simulink model "PTTransmCU"  (Simulink 7.5)
settings: Solver=ode45  StartTime=0.0  StopTime=inf  RelTol=1e-3
libraries: simulink x12, CarMaker4SL x1
(part 2 of 3)

== system PTTransmCU/CarMaker/IPG Vehicle/CarAndTrailer/Forces/Vehicle Forces ==
  Sync_In : Inport  OutDataType=sfix(16)  OutScaling=2^0
  Bus Creator1 : BusCreator  Inputs=12
  Bus Creator5 : BusCreator  Inputs=13
  Bus Creator8 : BusCreator  Inputs=16
  Demux : Demux  Outputs=16
  Demux1 : Demux  Outputs=12
  Demux5 : Demux  Outputs=13
  Forces : S-Function  FunctionName=CM_Sfun  Parameters='Forces'  EnableBusSupport=off
  Sync_Out : Outport  OutDataType=sfix(16)  OutScaling=2^0
  Car.Virtual : Outport  Port=2  OutDataType=sfix(16)  OutScaling=2^0
  Car.Aero : Outport  Port=3  OutDataType=sfix(16)  OutScaling=2^0
  Car.Load : Outport  Port=4  OutDataType=sfix(16)  OutScaling=2^0
  wires:
  Demux5/7 -> Bus Creator5/7  "car Aero vRes_1 z"
  Demux5/6 -> Bus Creator5/6  "car Aero vRes_1 y"
  Demux5/5 -> Bus Creator5/5  "car Aero vRes_1 x"
  Demux5/4 -> Bus Creator5/4  "Vehicle Wind_vel_0 z"
  Demux5/3 -> Bus Creator5/3  "Vehicle Wind_vel_0 y"
  Demux5/2 -> Bus Creator5/2  "Vehicle Wind_vel_0 x"
  Demux5/1 -> Bus Creator5/1  "Vehicle sRoadAero"
  Demux5/8 -> Bus Creator5/8  "car Aero Frc_1 x"
  Demux5/9 -> Bus Creator5/9  "car Aero Frc_1 y"
  Demux5/10 -> Bus Creator5/10  "car Aero Frc_1 z"
  Demux5/13 -> Bus Creator5/13  "car Aero Trq_1 z"
  Demux5/12 -> Bus Creator5/12  "car Aero Trq_1 y"
  Demux5/11 -> Bus Creator5/11  "car Aero Trq_1 x"
  Forces/4 -> Demux/1
  Demux/12 -> Bus Creator8/12  "Car Load_2 tz"
  Demux/11 -> Bus Creator8/11  "Car Load_2 ty"
  Demux/10 -> Bus Creator8/10  "Car Load_2 tx"
  Demux/9 -> Bus Creator8/9  "Car Load_2 mass"
  Demux/8 -> Bus Creator8/8  "Car Load_1 tz"
  Demux/7 -> Bus Creator8/7  "Car Load_1 ty"
  Demux/6 -> Bus Creator8/6  "Car Load_1 tx"
  Demux/5 -> Bus Creator8/5  "Car Load_1 mass"
  Demux/4 -> Bus Creator8/4  "Car Load_0 tz"
  Demux/3 -> Bus Creator8/3  "Car Load_0 ty"
  Demux/2 -> Bus Creator8/2  "Car Load_0 tx"
  Demux/1 -> Bus Creator8/1  "Car Load_0 mass"
  Bus Creator8/1 -> Car.Load/1
  Bus Creator1/1 -> Car.Virtual/1
  Forces/2 -> Demux1/1
  Forces/3 -> Demux5/1
  Demux1/3 -> Bus Creator1/3  "Car Virtual Frc_1 z"
  Demux1/2 -> Bus Creator1/2  "Car Virtual Frc_1 y"
  Demux1/1 -> Bus Creator1/1  "Car Virtual Frc_1 x"
  Bus Creator5/1 -> Car.Aero/1
  Forces/1 -> Sync_Out/1
  Sync_In/1 -> Forces/1
  Demux1/4 -> Bus Creator1/4  "Car Virtual Frc_0 x"
  Demux1/5 -> Bus Creator1/5  "Car Virtual Frc_0 y"
  Demux1/6 -> Bus Creator1/6  "Car Virtual Frc_0 z"
  Demux1/7 -> Bus Creator1/7  "Car Virtual Trq_1 x"
  Demux1/8 -> Bus Creator1/8  "Car Virtual Trq_1 y"
  Demux1/9 -> Bus Creator1/9  "Car Virtual Trq_1 z"
  Demux1/10 -> Bus Creator1/10  "Car Virtual Trq_0 x"
  Demux1/11 -> Bus Creator1/11  "Car Virtual Trq_0 y"
  Demux1/12 -> Bus Creator1/12  "Car Virtual Trq_0 z"
  Demux/13 -> Bus Creator8/13  "Car Load_3 mass"
  Demux/14 -> Bus Creator8/14  "Car Load_3 tx"
  Demux/15 -> Bus Creator8/15  "Car Load_3 ty"
  Demux/16 -> Bus Creator8/16  "Car Load_3 tz"

== system PTTransmCU/CarMaker/IPG Vehicle/CarAndTrailer/Trailer/CreateBus Car.Hitch.FrcTrq ==
  In1 : Inport  OutDataType=sfix(16)  OutScaling=2^0
  Bus Creator7 : BusCreator  Inputs=6
  Demux7 : Demux  Outputs=6
  Car.Hitch.FrcTrq : Outport  OutDataType=sfix(16)  OutScaling=2^0
  wires:
  Demux7/1 -> Bus Creator7/1  "Car Hitch Frc2Car x"
  Demux7/2 -> Bus Creator7/2  "Car Hitch Frc2Car y"
  Demux7/3 -> Bus Creator7/3  "Car Hitch Frc2Car z"
  Demux7/4 -> Bus Creator7/4  "Car Hitch Trq2Car x"
  Demux7/5 -> Bus Creator7/5  "Car Hitch Trq2Car y"
  Demux7/6 -> Bus Creator7/6  "Car Hitch Trq2Car z"
  Bus Creator7/1 -> Car.Hitch.FrcTrq/1
  In1/1 -> Demux7/1

== system PTTransmCU/CarMaker/IPG Vehicle/CarAndTrailer/Trailer/CreateBus Vhcl.Motion ==
  In1 : Inport  OutDataType=sfix(16)  OutScaling=2^0
  Demux1 : Demux  Outputs=16
  Mux1 : Mux  Inputs=16
  Out1 : Outport  OutDataType=sfix(16)  OutScaling=2^0
  wires:
  Mux1/1 -> Out1/1
  In1/1 -> Demux1/1
  Demux1/16 -> Mux1/16  "Vhcl YawAcc"
  Demux1/15 -> Mux1/15  "Vhcl YawRate"
  Demux1/14 -> Mux1/14  "Vhcl Yaw"
  Demux1/13 -> Mux1/13  "Vhcl PitchAcc"
  Demux1/12 -> Mux1/12  "Vhcl PitchVel"
  Demux1/11 -> Mux1/11  "Vhcl Pitch"
  Demux1/10 -> Mux1/10  "Vhcl RollAcc"
  Demux1/9 -> Mux1/9  "Vhcl RollVel"
  Demux1/8 -> Mux1/8  "Vhcl Roll"
  Demux1/7 -> Mux1/7  "Vhcl Hitch_Pos z"
  Demux1/6 -> Mux1/6  "Vhcl Hitch_Pos y"
  Demux1/5 -> Mux1/5  "Vhcl Hitch_Pos x"
  Demux1/4 -> Mux1/4  "Vhcl sRoadAero"
  Demux1/3 -> Mux1/3  "Vhcl sRoad"
  Demux1/2 -> Mux1/2  "Vhcl Distance"
  Demux1/1 -> Mux1/1  "Vhcl v"

== system PTTransmCU/CarMaker/IPG Vehicle/CarAndTrailer/Trailer/CreateBus Vhcl.PoI ==
  In1 : Inport  OutDataType=sfix(16)  OutScaling=2^0
  Bus Creator3 : BusCreator  Inputs=18
  Demux3 : Demux  Outputs=18
  Out1 : Outport  OutDataType=sfix(16)  OutScaling=2^0
  wires:
  Demux3/1 -> Bus Creator3/1  "Vhcl PoI_Pos x"
  Bus Creator3/1 -> Out1/1
  In1/1 -> Demux3/1
  Demux3/2 -> Bus Creator3/2  "Vhcl PoI_Pos y"
  Demux3/3 -> Bus Creator3/3  "Vhcl PoI_Pos z"
  Demux3/4 -> Bus Creator3/4  "Vhcl PoI_Vel x"
  Demux3/5 -> Bus Creator3/5  "Vhcl PoI_Vel y"
  Demux3/6 -> Bus Creator3/6  "Vhcl PoI_Vel z"
  Demux3/7 -> Bus Creator3/7  "Vhcl PoI_Acc x"
  Demux3/8 -> Bus Creator3/8  "Vhcl PoI_Acc y"
  Demux3/9 -> Bus Creator3/9  "Vhcl PoI_Acc z"
  Demux3/10 -> Bus Creator3/10  "Vhcl PoI_Vel_1 x"
  Demux3/11 -> Bus Creator3/11  "Vhcl PoI_Vel_1 y"
  Demux3/12 -> Bus Creator3/12  "Vhcl PoI_Vel_1 z"
  Demux3/13 -> Bus Creator3/13  "Vhcl PoI_Acc_1 x"
  Demux3/14 -> Bus Creator3/14  "Vhcl PoI_Acc_1 y"
  Demux3/15 -> Bus Creator3/15  "Vhcl PoI_Acc_1 z"
  Demux3/16 -> Bus Creator3/16  "Vhcl PoI_GCS Long"
  Demux3/17 -> Bus Creator3/17  "Vhcl PoI_GCS Lat"
  Demux3/18 -> Bus Creator3/18  "Vhcl PoI_GCS Elev"

== system PTTransmCU/CarMaker/IPG Vehicle/CarAndTrailer/Trailer/CreateBus Vhcl.Steering ==
  In1 : Inport  OutDataType=sfix(16)  OutScaling=2^0
  Bus Creator3 : BusCreator
  Demux : Demux
  Out1 : Outport  OutDataType=sfix(16)  OutScaling=2^0
  wires:
  In1/1 -> Demux/1
  Demux/4 -> Bus Creator3/4  "Vhcl Steering Trq"
  Demux/2 -> Bus Creator3/2  "Vhcl Steering AngVel"
  Demux/3 -> Bus Creator3/3  "Vhcl Steering AngAcc"
  Demux/1 -> Bus Creator3/1  "Vhcl Steering Ang"
  Bus Creator3/1 -> Out1/1

== system PTTransmCU/CarMaker/IPG Vehicle/CarAndTrailer/Trailer/CreateBus Vhcl.Wheel.FL ==
  In1 : Inport  OutDataType=sfix(16)  OutScaling=2^0
  Bus Creator3 : BusCreator  Inputs=14
  Demux3 : Demux  Outputs=14
  Out1 : Outport  OutDataType=sfix(16)  OutScaling=2^0
  wires:
  Demux3/1 -> Bus Creator3/1  "Vhcl Wheel FL t x"
  Bus Creator3/1 -> Out1/1
  In1/1 -> Demux3/1
  Demux3/2 -> Bus Creator3/2  "Vhcl Wheel FL t y"
  Demux3/3 -> Bus Creator3/3  "Vhcl Wheel FL t z"
  Demux3/4 -> Bus Creator3/4  "Vhcl Wheel FL r_zxy x"
  Demux3/5 -> Bus Creator3/5  "Vhcl Wheel FL r_zxy y"
  Demux3/6 -> Bus Creator3/6  "Vhcl Wheel FL r_zxy z"
  Demux3/7 -> Bus Creator3/7  "Vhcl Wheel FL Fx"
  Demux3/8 -> Bus Creator3/8  "Vhcl Wheel FL Fy"
  Demux3/9 -> Bus Creator3/9  "Vhcl Wheel FL Fz"
  Demux3/10 -> Bus Creator3/10  "Vhcl Wheel FL vBelt"
  Demux3/11 -> Bus Creator3/11  "Vhcl Wheel FL LongSlip"
  Demux3/12 -> Bus Creator3/12  "Vhcl Wheel FL SideSlip"
  Demux3/13 -> Bus Creator3/13  "Vhcl Wheel FL Trq_T2W"
  Demux3/14 -> Bus Creator3/14  "Vhcl Wheel FL Trq_WhlBearing"

== system PTTransmCU/CarMaker/IPG Vehicle/CarAndTrailer/Trailer/CreateBus Vhcl.Wheel.FR ==
  In1 : Inport  OutDataType=sfix(16)  OutScaling=2^0
  Bus Creator3 : BusCreator  Inputs=14
  Demux3 : Demux  Outputs=14
  Out1 : Outport  OutDataType=sfix(16)  OutScaling=2^0
  wires:
  Demux3/1 -> Bus Creator3/1  "Vhcl Wheel FR t x"
  Bus Creator3/1 -> Out1/1
  In1/1 -> Demux3/1
  Demux3/2 -> Bus Creator3/2  "Vhcl Wheel FR t y"
  Demux3/3 -> Bus Creator3/3  "Vhcl Wheel FR t z"
  Demux3/4 -> Bus Creator3/4  "Vhcl Wheel FR r_zxy x"
  Demux3/5 -> Bus Creator3/5  "Vhcl Wheel FR r_zxy y"
  Demux3/6 -> Bus Creator3/6  "Vhcl Wheel FR r_zxy z"
  Demux3/7 -> Bus Creator3/7  "Vhcl Wheel FR Fx"
  Demux3/8 -> Bus Creator3/8  "Vhcl Wheel FR Fy"
  Demux3/9 -> Bus Creator3/9  "Vhcl Wheel FR Fz"
  Demux3/10 -> Bus Creator3/10  "Vhcl Wheel FR vBelt"
  Demux3/11 -> Bus Creator3/11  "Vhcl Wheel FR LongSlip"
  Demux3/12 -> Bus Creator3/12  "Vhcl Wheel FR SideSlip"
  Demux3/13 -> Bus Creator3/13  "Vhcl Wheel FR Trq_T2W"
  Demux3/14 -> Bus Creator3/14  "Vhcl Wheel FR Trq_WhlBearing"

== system PTTransmCU/CarMaker/IPG Vehicle/CarAndTrailer/Trailer/CreateBus Vhcl.Wheel.RL ==
  In1 : Inport  OutDataType=sfix(16)  OutScaling=2^0
  Bus Creator3 : BusCreator  Inputs=14
  Demux3 : Demux  Outputs=14
  Out1 : Outport  OutDataType=sfix(16)  OutScaling=2^0
  wires:
  Demux3/1 -> Bus Creator3/1  "Vhcl Wheel RL t x"
  Bus Creator3/1 -> Out1/1
  In1/1 -> Demux3/1
  Demux3/2 -> Bus Creator3/2  "Vhcl Wheel RL t y"
  Demux3/3 -> Bus Creator3/3  "Vhcl Wheel RL t z"
  Demux3/4 -> Bus Creator3/4  "Vhcl Wheel RL r_zxy x"
  Demux3/5 -> Bus Creator3/5  "Vhcl Wheel RL r_zxy y"
  Demux3/6 -> Bus Creator3/6  "Vhcl Wheel RL r_zxy z"
  Demux3/7 -> Bus Creator3/7  "Vhcl Wheel RL Fx"
  Demux3/8 -> Bus Creator3/8  "Vhcl Wheel RL Fy"
  Demux3/9 -> Bus Creator3/9  "Vhcl Wheel RL Fz"
  Demux3/10 -> Bus Creator3/10  "Vhcl Wheel RL vBelt"
  Demux3/11 -> Bus Creator3/11  "Vhcl Wheel RL LongSlip"
  Demux3/12 -> Bus Creator3/12  "Vhcl Wheel RL SideSlip"
  Demux3/13 -> Bus Creator3/13  "Vhcl Wheel RL Trq_T2W"
  Demux3/14 -> Bus Creator3/14  "Vhcl Wheel RL Trq_WhlBearing"

== system PTTransmCU/CarMaker/IPG Vehicle/CarAndTrailer/Trailer/CreateBus Vhcl.Wheel.RR ==
  In1 : Inport  OutDataType=sfix(16)  OutScaling=2^0
  Bus Creator3 : BusCreator  Inputs=14
  Demux3 : Demux  Outputs=14
  Out1 : Outport  OutDataType=sfix(16)  OutScaling=2^0
  wires:
  Demux3/1 -> Bus Creator3/1  "Vhcl Wheel RR t x"
  Bus Creator3/1 -> Out1/1
  In1/1 -> Demux3/1
  Demux3/2 -> Bus Creator3/2  "Vhcl Wheel RR t y"
  Demux3/3 -> Bus Creator3/3  "Vhcl Wheel RR t z"
  Demux3/4 -> Bus Creator3/4  "Vhcl Wheel RR r_zxy x"
  Demux3/5 -> Bus Creator3/5  "Vhcl Wheel RR r_zxy y"
  Demux3/6 -> Bus Creator3/6  "Vhcl Wheel RR r_zxy z"
  Demux3/7 -> Bus Creator3/7  "Vhcl Wheel RR Fx"
  Demux3/8 -> Bus Creator3/8  "Vhcl Wheel RR Fy"
  Demux3/9 -> Bus Creator3/9  "Vhcl Wheel RR Fz"
  Demux3/10 -> Bus Creator3/10  "Vhcl Wheel RR vBelt"
  Demux3/11 -> Bus Creator3/11  "Vhcl Wheel RR LongSlip"
  Demux3/12 -> Bus Creator3/12  "Vhcl Wheel RR SideSlip"
  Demux3/13 -> Bus Creator3/13  "Vhcl Wheel RR Trq_T2W"
  Demux3/14 -> Bus Creator3/14  "Vhcl Wheel RR Trq_WhlBearing"

== system PTTransmCU/CarMaker/IPG Vehicle/PowerTrain/TCU Example/CreateBus TCU ClutchOut ==
  In : Inport
  BusCreator : BusCreator  Inputs=1
  Demux : Demux  Outputs=1
  Out : Outport
  wires:
  In/1 -> Demux/1
  BusCreator/1 -> Out/1
  Demux/1 -> BusCreator/1  "TCU ClutchOut Pos"

== system PTTransmCU/CarMaker/IPG Vehicle/PowerTrain/TCU Example/CreateBus TCU GearBoxM_Out0 ==
  In : Inport
  BusCreator : BusCreator
  Demux : Demux
  Out : Outport
  wires:
  In/1 -> Demux/1
  BusCreator/1 -> Out/1
  Demux/1 -> BusCreator/1  "TCU GearBoxM_Out0 GearNoTrg"
  Demux/2 -> BusCreator/2  "TCU GearBoxM_Out0 set_ParkBrake"
  Demux/3 -> BusCreator/3  "TCU GearBoxM_Out0 Trq_in_off"
  Demux/4 -> BusCreator/4  "TCU GearBoxM_Out0 Clutch Pos"

== system PTTransmCU/CarMaker/IPG Vehicle/PowerTrain/TCU Example/CreateBus TCU GearBoxM_Out1 ==
  In : Inport
  BusCreator : BusCreator
  Demux : Demux
  Out : Outport
  wires:
  In/1 -> Demux/1
  BusCreator/1 -> Out/1
  Demux/1 -> BusCreator/1  "TCU GearBoxM_Out1 GearNoTrg"
  Demux/2 -> BusCreator/2  "TCU GearBoxM_Out1 set_ParkBrake"
  Demux/3 -> BusCreator/3  "TCU GearBoxM_Out1 Trq_in_off"
  Demux/4 -> BusCreator/4  "TCU GearBoxM_Out1 Clutch Pos"

== system PTTransmCU/CarMaker/IPG Vehicle/PowerTrain/TCU Example/CreateBus TCU GearBoxM_Out2 ==
  In : Inport
  BusCreator : BusCreator
  Demux : Demux
  Out : Outport
  wires:
  In/1 -> Demux/1
  BusCreator/1 -> Out/1
  Demux/1 -> BusCreator/1  "TCU GearBoxM_Out2 GearNoTrg"
  Demux/2 -> BusCreator/2  "TCU GearBoxM_Out2 set_ParkBrake"
  Demux/3 -> BusCreator/3  "TCU GearBoxM_Out2 Trq_in_off"
  Demux/4 -> BusCreator/4  "TCU GearBoxM_Out2 Clutch Pos"

== system PTTransmCU/CarMaker/IPG Vehicle/PowerTrain/TCU Example/CreateBus TCU GearBoxM_Out3 ==
  In : Inport
  BusCreator : BusCreator
  Demux : Demux
  Out : Outport
  wires:
  In/1 -> Demux/1
  BusCreator/1 -> Out/1
  Demux/1 -> BusCreator/1  "TCU GearBoxM_Out3 GearNoTrg"
  Demux/2 -> BusCreator/2  "TCU GearBoxM_Out3 set_ParkBrake"
  Demux/3 -> BusCreator/3  "TCU GearBoxM_Out3 Trq_in_off"
  Demux/4 -> BusCreator/4  "TCU GearBoxM_Out3 Clutch Pos"

== system PTTransmCU/CarMaker/IPG Vehicle/PowerTrain/TCU Example/CreateBus TCU GearBoxOut ==
  In : Inport
  BusCreator : BusCreator
  Demux : Demux
  Out : Outport
  wires:
  In/1 -> Demux/1
  BusCreator/1 -> Out/1
  Demux/1 -> BusCreator/1  "TCU GearBoxOut GearNoTrg"
  Demux/2 -> BusCreator/2  "TCU GearBoxOut set_ParkBrake"
  Demux/3 -> BusCreator/3  "TCU GearBoxOut Trq_in_off"
  Demux/4 -> BusCreator/4  "TCU GearBoxOut Clutch Pos"

== system PTTransmCU/CarMaker/IPG Vehicle/PowerTrain/TCU Example/CreateBus TCU Status ==
  In : Inport
  BusCreator : BusCreator  Inputs=1
  Demux : Demux  Outputs=1
  Out : Outport
  wires:
  In/1 -> Demux/1
  BusCreator/1 -> Out/1
  Demux/1 -> BusCreator/1  "TCU_Out Status"

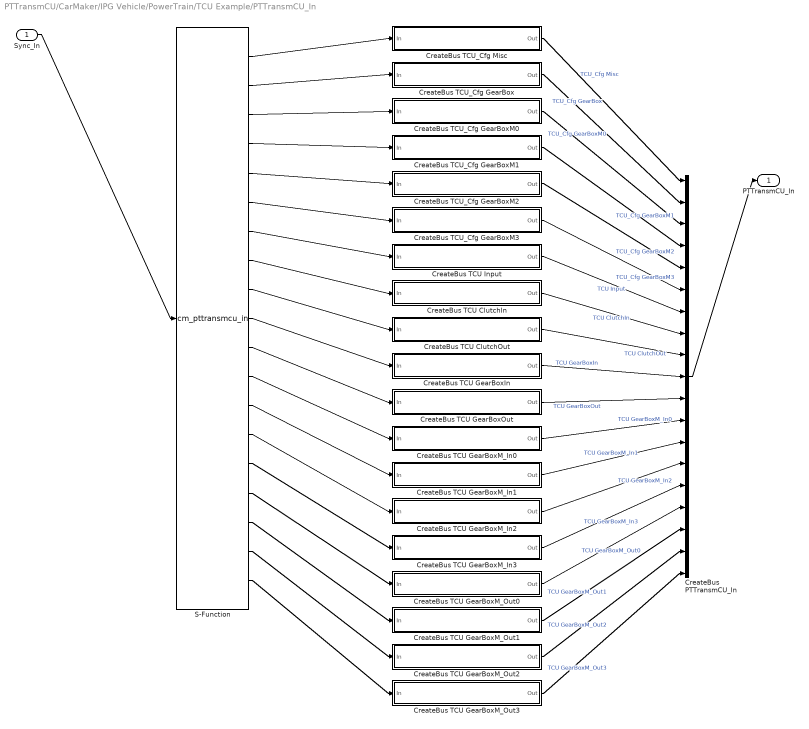
== system PTTransmCU/CarMaker/IPG Vehicle/PowerTrain/TCU Example/PTTransmCU_In ==
  Sync_In : Inport
  CreateBus PTTransmCU_In : BusCreator  Inputs=19
  CreateBus TCU ClutchIn : Subsystem
  CreateBus TCU ClutchOut : Subsystem
  CreateBus TCU GearBoxIn : Subsystem
  CreateBus TCU GearBoxM_In0 : Subsystem
  CreateBus TCU GearBoxM_In1 : Subsystem
  CreateBus TCU GearBoxM_In2 : Subsystem
  CreateBus TCU GearBoxM_In3 : Subsystem
  CreateBus TCU GearBoxM_Out0 : Subsystem
  CreateBus TCU GearBoxM_Out1 : Subsystem
  CreateBus TCU GearBoxM_Out2 : Subsystem
  CreateBus TCU GearBoxM_Out3 : Subsystem
  CreateBus TCU GearBoxOut : Subsystem
  CreateBus TCU Input : Subsystem
  CreateBus TCU_Cfg GearBox : Subsystem
  CreateBus TCU_Cfg GearBoxM0 : Subsystem
  CreateBus TCU_Cfg GearBoxM1 : Subsystem
  CreateBus TCU_Cfg GearBoxM2 : Subsystem
  CreateBus TCU_Cfg GearBoxM3 : Subsystem
  CreateBus TCU_Cfg Misc : Subsystem
  S-Function : S-Function  FunctionName=cm_pttransmcu_in  EnableBusSupport=off
  PTTransmCU_In : Outport
  wires:
  Sync_In/1 -> S-Function/1
  CreateBus PTTransmCU_In/1 -> PTTransmCU_In/1
  S-Function/1 -> CreateBus TCU_Cfg Misc/1(In)
  CreateBus TCU_Cfg Misc/1(Out) -> CreateBus PTTransmCU_In/1  "TCU_Cfg Misc"
  S-Function/2 -> CreateBus TCU_Cfg GearBox/1(In)
  CreateBus TCU_Cfg GearBox/1(Out) -> CreateBus PTTransmCU_In/2  "TCU_Cfg GearBox"
  S-Function/3 -> CreateBus TCU_Cfg GearBoxM0/1(In)
  CreateBus TCU_Cfg GearBoxM0/1(Out) -> CreateBus PTTransmCU_In/3  "TCU_Cfg GearBoxM0"
  S-Function/4 -> CreateBus TCU_Cfg GearBoxM1/1(In)
  CreateBus TCU_Cfg GearBoxM1/1(Out) -> CreateBus PTTransmCU_In/4  "TCU_Cfg GearBoxM1"
  S-Function/5 -> CreateBus TCU_Cfg GearBoxM2/1(In)
  CreateBus TCU_Cfg GearBoxM2/1(Out) -> CreateBus PTTransmCU_In/5  "TCU_Cfg GearBoxM2"
  S-Function/6 -> CreateBus TCU_Cfg GearBoxM3/1(In)
  CreateBus TCU_Cfg GearBoxM3/1(Out) -> CreateBus PTTransmCU_In/6  "TCU_Cfg GearBoxM3"
  S-Function/7 -> CreateBus TCU Input/1(In)
  CreateBus TCU Input/1(Out) -> CreateBus PTTransmCU_In/7  "TCU Input"
  S-Function/8 -> CreateBus TCU ClutchIn/1(In)
  CreateBus TCU ClutchIn/1(Out) -> CreateBus PTTransmCU_In/8  "TCU ClutchIn"
  S-Function/9 -> CreateBus TCU ClutchOut/1(In)
  CreateBus TCU ClutchOut/1(Out) -> CreateBus PTTransmCU_In/9  "TCU ClutchOut"
  S-Function/10 -> CreateBus TCU GearBoxIn/1(In)
  CreateBus TCU GearBoxIn/1(Out) -> CreateBus PTTransmCU_In/10  "TCU GearBoxIn"
  S-Function/11 -> CreateBus TCU GearBoxOut/1(In)
  CreateBus TCU GearBoxOut/1(Out) -> CreateBus PTTransmCU_In/11  "TCU GearBoxOut"
  S-Function/12 -> CreateBus TCU GearBoxM_In0/1(In)
  CreateBus TCU GearBoxM_In0/1(Out) -> CreateBus PTTransmCU_In/12  "TCU GearBoxM_In0"
  S-Function/13 -> CreateBus TCU GearBoxM_In1/1(In)
  CreateBus TCU GearBoxM_In1/1(Out) -> CreateBus PTTransmCU_In/13  "TCU GearBoxM_In1"
  S-Function/14 -> CreateBus TCU GearBoxM_In2/1(In)
  CreateBus TCU GearBoxM_In2/1(Out) -> CreateBus PTTransmCU_In/14  "TCU GearBoxM_In2"
  S-Function/15 -> CreateBus TCU GearBoxM_In3/1(In)
  CreateBus TCU GearBoxM_In3/1(Out) -> CreateBus PTTransmCU_In/15  "TCU GearBoxM_In3"
  S-Function/16 -> CreateBus TCU GearBoxM_Out0/1(In)
  CreateBus TCU GearBoxM_Out0/1(Out) -> CreateBus PTTransmCU_In/16  "TCU GearBoxM_Out0"
  S-Function/17 -> CreateBus TCU GearBoxM_Out1/1(In)
  CreateBus TCU GearBoxM_Out1/1(Out) -> CreateBus PTTransmCU_In/17  "TCU GearBoxM_Out1"
  S-Function/18 -> CreateBus TCU GearBoxM_Out2/1(In)
  CreateBus TCU GearBoxM_Out2/1(Out) -> CreateBus PTTransmCU_In/18  "TCU GearBoxM_Out2"
  S-Function/19 -> CreateBus TCU GearBoxM_Out3/1(In)
  CreateBus TCU GearBoxM_Out3/1(Out) -> CreateBus PTTransmCU_In/19  "TCU GearBoxM_Out3"

== system PTTransmCU/CarMaker/IPG Vehicle/PowerTrain/TCU Example/PTTransmCU_Out ==
  TCU Status : Inport
  TCU ClutchOut : Inport  Port=2
  TCU GearBoxOut : Inport  Port=3
  TCU GearBoxM_Out0 : Inport  Port=4
  TCU GearBoxM_Out1 : Inport  Port=5
  TCU GearBoxM_Out2 : Inport  Port=6
  TCU GearBoxM_Out3 : Inport  Port=7
  S-Function : S-Function  FunctionName=cm_pttransmcu_out  EnableBusSupport=off
  wires:
  TCU Status/1 -> S-Function/1
  TCU ClutchOut/1 -> S-Function/2
  TCU GearBoxOut/1 -> S-Function/3
  TCU GearBoxM_Out0/1 -> S-Function/4
  TCU GearBoxM_Out1/1 -> S-Function/5
  TCU GearBoxM_Out2/1 -> S-Function/6
  TCU GearBoxM_Out3/1 -> S-Function/7

== system PTTransmCU/CarMaker/IPG Vehicle/PowerTrain/TCU Example/TCU Example ==
  note: PTTransmCU model MyTransmCU example, that only works with
      | the 'Generic' powertrain and the 'Manual' gearbox.
  TCUIn : Inport  OutDataType=sfix(16)  OutScaling=2^0
  Bus Creator : BusCreator  Inputs=2
  Bus Selector : BusSelector  OutputSignals=TCU GearBoxIn GearNoTrg
  Bus Selector1 : BusSelector  OutputSignals=TCU Input.TCU Ignition,TCU GearBoxIn.TCU GearBoxIn GearNo,TCU GearBoxOut,TCU ClutchOut,TCU_Cfg GearBox.TCU_Cfg GearBox nFGears,TCU_Cfg GearBox.TCU_Cfg GearBox nBGears
  Bus Selector2 : BusSelector  OutputSignals=TCU GearBoxIn GearNoTrg,TCU GearBoxIn set_ParkBrake,TCU GearBoxIn Clutch Pos
  Don't do anything : Subsystem  TreatAsAtomicUnit=on
  If : If  NumInputs=3  IfExpression=~u1  ElseIfExpressions=u2 == u3
  If Action Subsystem2 : Subsystem  TreatAsAtomicUnit=on
  Merge1 : Merge  Inputs=3
  Merge2 : Merge  Inputs=3  InitialOutput=0
  Retrun Zero : Subsystem  TreatAsAtomicUnit=on
  ClutchOut.Pos : Outport  OutDataType=sfix(16)  OutScaling=2^0
  GearBoxOut.GearNoTrg : Outport  Port=2  OutDataType=sfix(16)  OutScaling=2^0
  GearBoxOut.set_ParkBrake : Outport  Port=3  OutDataType=sfix(16)  OutScaling=2^0
  GearBoxOut.Clutch.Pos : Outport  Port=4  OutDataType=sfix(16)  OutScaling=2^0
  wires:
  TCUIn/1 -> Bus Selector1/1
  If/1 -> Retrun Zero/Action
  Bus Selector1/2 -> If/2, If Action Subsystem2/4(GearNo)  "<TCU GearBoxIn GearNo>"
  Bus Selector/1 -> If/3  "<TCU GearBoxIn GearNoTrg>"
  If/2 -> Don't do anything/Action
  If/3 -> If Action Subsystem2/Action
  Bus Selector1/5 -> Bus Creator/1  "<TCU_Cfg GearBox nFGears>"
  Bus Selector1/6 -> Bus Creator/2  "<TCU_Cfg GearBox nBGears>"
  Bus Creator/1 -> If Action Subsystem2/3(CfgIF)
  Retrun Zero/2(ClutchOut.Pos) -> Merge1/1
  Don't do anything/2(ClutchOut.Pos) -> Merge1/2
  If Action Subsystem2/2(ClutchOut.Pos) -> Merge1/3
  Retrun Zero/1(GearBoxOut1) -> Merge2/1
  Don't do anything/1(GearBoxOut1) -> Merge2/2
  If Action Subsystem2/1(GearBoxOut1) -> Merge2/3
  Merge2/1 -> Bus Selector2/1
  Bus Selector1/3 -> Bus Selector/1, Retrun Zero/1(GearBoxOut), Don't do anything/1(GearBoxOut), If Action Subsystem2/1(GearBoxOut)  "<TCU GearBoxOut>"
  Bus Selector1/4 -> Don't do anything/2(ClutchOut), If Action Subsystem2/2(ClutchOut)  "<TCU ClutchOut>"
  Merge1/1 -> ClutchOut.Pos/1
  Bus Selector1/1 -> If/1  "<TCU Ignition>"
  Bus Selector2/1 -> GearBoxOut.GearNoTrg/1  "<TCU GearBoxIn GearNoTrg>"
  Bus Selector2/2 -> GearBoxOut.set_ParkBrake/1  "<TCU GearBoxIn set_ParkBrake>"
  Bus Selector2/3 -> GearBoxOut.Clutch.Pos/1  "<TCU GearBoxIn Clutch Pos>"

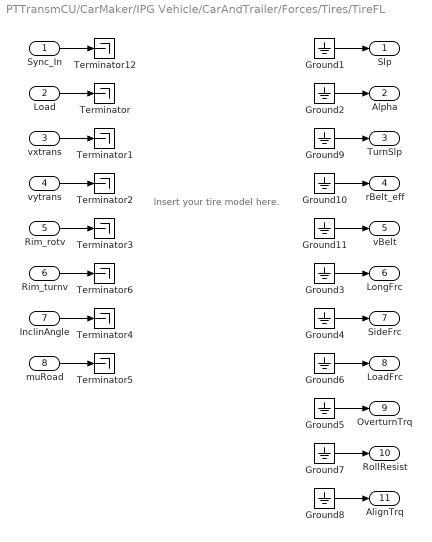
== system PTTransmCU/CarMaker/IPG Vehicle/CarAndTrailer/Forces/Tires/TireFL ==
  note: Insert your tire model here.
  Sync_In : Inport  OutDataType=sfix(16)  OutScaling=2^0
  Load : Inport  Port=2  OutDataType=sfix(16)  OutScaling=2^0
  vxtrans : Inport  Port=3  OutDataType=sfix(16)  OutScaling=2^0
  vytrans : Inport  Port=4  OutDataType=sfix(16)  OutScaling=2^0
  Rim_rotv : Inport  Port=5  OutDataType=sfix(16)  OutScaling=2^0
  Rim_turnv : Inport  Port=6  OutDataType=sfix(16)  OutScaling=2^0
  InclinAngle : Inport  Port=7  OutDataType=sfix(16)  OutScaling=2^0
  muRoad : Inport  Port=8  OutDataType=sfix(16)  OutScaling=2^0
  Ground{1..11} (11 alike) : Ground
  Terminator{,1..6,12} (8 alike) : Terminator
  Slp : Outport  OutDataType=sfix(16)  OutScaling=2^0
  Alpha : Outport  Port=2  OutDataType=sfix(16)  OutScaling=2^0
  TurnSlp : Outport  Port=3  OutDataType=sfix(16)  OutScaling=2^0
  rBelt_eff : Outport  Port=4  OutDataType=sfix(16)  OutScaling=2^0
  vBelt : Outport  Port=5  OutDataType=sfix(16)  OutScaling=2^0
  LongFrc : Outport  Port=6  OutDataType=sfix(16)  OutScaling=2^0
  SideFrc : Outport  Port=7  OutDataType=sfix(16)  OutScaling=2^0
  LoadFrc : Outport  Port=8  OutDataType=sfix(16)  OutScaling=2^0
  OverturnTrq : Outport  Port=9  OutDataType=sfix(16)  OutScaling=2^0
  RollResist : Outport  Port=10  OutDataType=sfix(16)  OutScaling=2^0
  AlignTrq : Outport  Port=11  OutDataType=sfix(16)  OutScaling=2^0
  wires:
  Ground8/1 -> AlignTrq/1
  Ground7/1 -> RollResist/1
  Ground6/1 -> LoadFrc/1
  Ground1/1 -> Slp/1
  Load/1 -> Terminator/1
  muRoad/1 -> Terminator5/1
  InclinAngle/1 -> Terminator4/1
  Rim_rotv/1 -> Terminator3/1
  vytrans/1 -> Terminator2/1
  vxtrans/1 -> Terminator1/1
  Ground5/1 -> OverturnTrq/1
  Ground4/1 -> SideFrc/1
  Ground3/1 -> LongFrc/1
  Ground2/1 -> Alpha/1
  Sync_In/1 -> Terminator12/1
  Rim_turnv/1 -> Terminator6/1
  Ground9/1 -> TurnSlp/1
  Ground10/1 -> rBelt_eff/1
  Ground11/1 -> vBelt/1

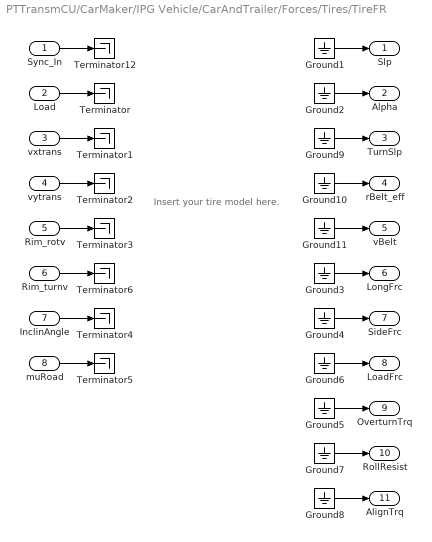
== system PTTransmCU/CarMaker/IPG Vehicle/CarAndTrailer/Forces/Tires/TireFR ==
  note: Insert your tire model here.
  Sync_In : Inport  OutDataType=sfix(16)  OutScaling=2^0
  Load : Inport  Port=2  OutDataType=sfix(16)  OutScaling=2^0
  vxtrans : Inport  Port=3  OutDataType=sfix(16)  OutScaling=2^0
  vytrans : Inport  Port=4  OutDataType=sfix(16)  OutScaling=2^0
  Rim_rotv : Inport  Port=5  OutDataType=sfix(16)  OutScaling=2^0
  Rim_turnv : Inport  Port=6  OutDataType=sfix(16)  OutScaling=2^0
  InclinAngle : Inport  Port=7  OutDataType=sfix(16)  OutScaling=2^0
  muRoad : Inport  Port=8  OutDataType=sfix(16)  OutScaling=2^0
  Ground{1..11} (11 alike) : Ground
  Terminator{,1..6,12} (8 alike) : Terminator
  Slp : Outport  OutDataType=sfix(16)  OutScaling=2^0
  Alpha : Outport  Port=2  OutDataType=sfix(16)  OutScaling=2^0
  TurnSlp : Outport  Port=3  OutDataType=sfix(16)  OutScaling=2^0
  rBelt_eff : Outport  Port=4  OutDataType=sfix(16)  OutScaling=2^0
  vBelt : Outport  Port=5  OutDataType=sfix(16)  OutScaling=2^0
  LongFrc : Outport  Port=6  OutDataType=sfix(16)  OutScaling=2^0
  SideFrc : Outport  Port=7  OutDataType=sfix(16)  OutScaling=2^0
  LoadFrc : Outport  Port=8  OutDataType=sfix(16)  OutScaling=2^0
  OverturnTrq : Outport  Port=9  OutDataType=sfix(16)  OutScaling=2^0
  RollResist : Outport  Port=10  OutDataType=sfix(16)  OutScaling=2^0
  AlignTrq : Outport  Port=11  OutDataType=sfix(16)  OutScaling=2^0
  wires:
  Ground8/1 -> AlignTrq/1
  Ground7/1 -> RollResist/1
  Ground6/1 -> LoadFrc/1
  Ground1/1 -> Slp/1
  Load/1 -> Terminator/1
  muRoad/1 -> Terminator5/1
  InclinAngle/1 -> Terminator4/1
  Rim_rotv/1 -> Terminator3/1
  vytrans/1 -> Terminator2/1
  vxtrans/1 -> Terminator1/1
  Ground5/1 -> OverturnTrq/1
  Ground4/1 -> SideFrc/1
  Ground3/1 -> LongFrc/1
  Ground2/1 -> Alpha/1
  Sync_In/1 -> Terminator12/1
  Rim_turnv/1 -> Terminator6/1
  Ground9/1 -> TurnSlp/1
  Ground10/1 -> rBelt_eff/1
  Ground11/1 -> vBelt/1

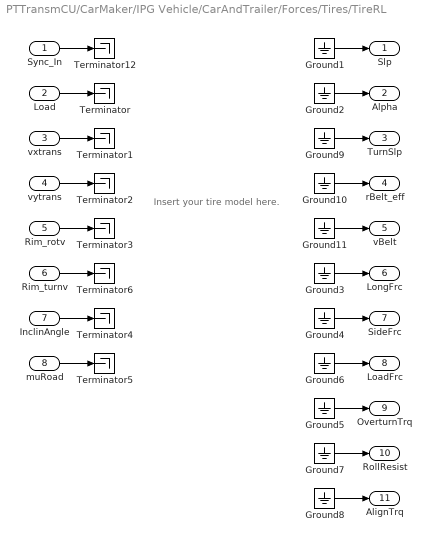
== system PTTransmCU/CarMaker/IPG Vehicle/CarAndTrailer/Forces/Tires/TireRL ==
  note: Insert your tire model here.
  Sync_In : Inport  OutDataType=sfix(16)  OutScaling=2^0
  Load : Inport  Port=2  OutDataType=sfix(16)  OutScaling=2^0
  vxtrans : Inport  Port=3  OutDataType=sfix(16)  OutScaling=2^0
  vytrans : Inport  Port=4  OutDataType=sfix(16)  OutScaling=2^0
  Rim_rotv : Inport  Port=5  OutDataType=sfix(16)  OutScaling=2^0
  Rim_turnv : Inport  Port=6  OutDataType=sfix(16)  OutScaling=2^0
  InclinAngle : Inport  Port=7  OutDataType=sfix(16)  OutScaling=2^0
  muRoad : Inport  Port=8  OutDataType=sfix(16)  OutScaling=2^0
  Ground{1..11} (11 alike) : Ground
  Terminator{,1..6,12} (8 alike) : Terminator
  Slp : Outport  OutDataType=sfix(16)  OutScaling=2^0
  Alpha : Outport  Port=2  OutDataType=sfix(16)  OutScaling=2^0
  TurnSlp : Outport  Port=3  OutDataType=sfix(16)  OutScaling=2^0
  rBelt_eff : Outport  Port=4  OutDataType=sfix(16)  OutScaling=2^0
  vBelt : Outport  Port=5  OutDataType=sfix(16)  OutScaling=2^0
  LongFrc : Outport  Port=6  OutDataType=sfix(16)  OutScaling=2^0
  SideFrc : Outport  Port=7  OutDataType=sfix(16)  OutScaling=2^0
  LoadFrc : Outport  Port=8  OutDataType=sfix(16)  OutScaling=2^0
  OverturnTrq : Outport  Port=9  OutDataType=sfix(16)  OutScaling=2^0
  RollResist : Outport  Port=10  OutDataType=sfix(16)  OutScaling=2^0
  AlignTrq : Outport  Port=11  OutDataType=sfix(16)  OutScaling=2^0
  wires:
  Ground8/1 -> AlignTrq/1
  Ground7/1 -> RollResist/1
  Ground6/1 -> LoadFrc/1
  Ground1/1 -> Slp/1
  Load/1 -> Terminator/1
  muRoad/1 -> Terminator5/1
  InclinAngle/1 -> Terminator4/1
  Rim_rotv/1 -> Terminator3/1
  vytrans/1 -> Terminator2/1
  vxtrans/1 -> Terminator1/1
  Ground5/1 -> OverturnTrq/1
  Ground4/1 -> SideFrc/1
  Ground3/1 -> LongFrc/1
  Ground2/1 -> Alpha/1
  Sync_In/1 -> Terminator12/1
  Rim_turnv/1 -> Terminator6/1
  Ground9/1 -> TurnSlp/1
  Ground10/1 -> rBelt_eff/1
  Ground11/1 -> vBelt/1

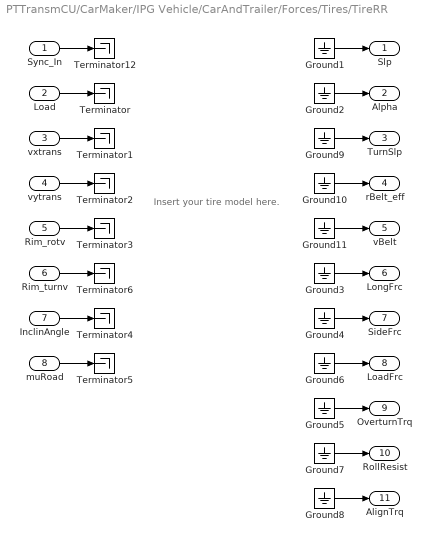
== system PTTransmCU/CarMaker/IPG Vehicle/CarAndTrailer/Forces/Tires/TireRR ==
  note: Insert your tire model here.
  Sync_In : Inport  OutDataType=sfix(16)  OutScaling=2^0
  Load : Inport  Port=2  OutDataType=sfix(16)  OutScaling=2^0
  vxtrans : Inport  Port=3  OutDataType=sfix(16)  OutScaling=2^0
  vytrans : Inport  Port=4  OutDataType=sfix(16)  OutScaling=2^0
  Rim_rotv : Inport  Port=5  OutDataType=sfix(16)  OutScaling=2^0
  Rim_turnv : Inport  Port=6  OutDataType=sfix(16)  OutScaling=2^0
  InclinAngle : Inport  Port=7  OutDataType=sfix(16)  OutScaling=2^0
  muRoad : Inport  Port=8  OutDataType=sfix(16)  OutScaling=2^0
  Ground{1..11} (11 alike) : Ground
  Terminator{,1..6,12} (8 alike) : Terminator
  Slp : Outport  OutDataType=sfix(16)  OutScaling=2^0
  Alpha : Outport  Port=2  OutDataType=sfix(16)  OutScaling=2^0
  TurnSlp : Outport  Port=3  OutDataType=sfix(16)  OutScaling=2^0
  rBelt_eff : Outport  Port=4  OutDataType=sfix(16)  OutScaling=2^0
  vBelt : Outport  Port=5  OutDataType=sfix(16)  OutScaling=2^0
  LongFrc : Outport  Port=6  OutDataType=sfix(16)  OutScaling=2^0
  SideFrc : Outport  Port=7  OutDataType=sfix(16)  OutScaling=2^0
  LoadFrc : Outport  Port=8  OutDataType=sfix(16)  OutScaling=2^0
  OverturnTrq : Outport  Port=9  OutDataType=sfix(16)  OutScaling=2^0
  RollResist : Outport  Port=10  OutDataType=sfix(16)  OutScaling=2^0
  AlignTrq : Outport  Port=11  OutDataType=sfix(16)  OutScaling=2^0
  wires:
  Ground8/1 -> AlignTrq/1
  Ground7/1 -> RollResist/1
  Ground6/1 -> LoadFrc/1
  Ground1/1 -> Slp/1
  Load/1 -> Terminator/1
  muRoad/1 -> Terminator5/1
  InclinAngle/1 -> Terminator4/1
  Rim_rotv/1 -> Terminator3/1
  vytrans/1 -> Terminator2/1
  vxtrans/1 -> Terminator1/1
  Ground5/1 -> OverturnTrq/1
  Ground4/1 -> SideFrc/1
  Ground3/1 -> LongFrc/1
  Ground2/1 -> Alpha/1
  Sync_In/1 -> Terminator12/1
  Rim_turnv/1 -> Terminator6/1
  Ground9/1 -> TurnSlp/1
  Ground10/1 -> rBelt_eff/1
  Ground11/1 -> vBelt/1

== system PTTransmCU/CarMaker/IPG Vehicle/PowerTrain/TCU Example/PTTransmCU_In/CreateBus TCU ClutchIn ==
  In : Inport
  BusCreator : BusCreator  Inputs=7
  Demux : Demux  Outputs=7
  Out : Outport
  wires:
  In/1 -> Demux/1
  BusCreator/1 -> Out/1
  Demux/1 -> BusCreator/1  "TCU ClutchIn rotv_in"
  Demux/2 -> BusCreator/2  "TCU ClutchIn rotv_out"
  Demux/3 -> BusCreator/3  "TCU ClutchIn rotv_out_trg"
  Demux/4 -> BusCreator/4  "TCU ClutchIn Trq_in"
  Demux/5 -> BusCreator/5  "TCU ClutchIn Trq_out"
  Demux/6 -> BusCreator/6  "TCU ClutchIn Trq_out_trg"
  Demux/7 -> BusCreator/7  "TCU ClutchIn i_TrqIn2Out"

== system PTTransmCU/CarMaker/IPG Vehicle/PowerTrain/TCU Example/PTTransmCU_In/CreateBus TCU ClutchOut ==
  In : Inport
  BusCreator : BusCreator  Inputs=1
  Demux : Demux  Outputs=1
  Out : Outport
  wires:
  In/1 -> Demux/1
  BusCreator/1 -> Out/1
  Demux/1 -> BusCreator/1  "TCU ClutchOut Pos"

== system PTTransmCU/CarMaker/IPG Vehicle/PowerTrain/TCU Example/PTTransmCU_In/CreateBus TCU GearBoxIn ==
  In : Inport
  BusCreator : BusCreator  Inputs=15
  Demux : Demux  Outputs=15
  Out : Outport
  wires:
  In/1 -> Demux/1
  BusCreator/1 -> Out/1
  Demux/1 -> BusCreator/1  "TCU GearBoxIn GearNo"
  Demux/2 -> BusCreator/2  "TCU GearBoxIn i"
  Demux/3 -> BusCreator/3  "TCU GearBoxIn rotv_in"
  Demux/4 -> BusCreator/4  "TCU GearBoxIn rotv_in_trg"
  Demux/5 -> BusCreator/5  "TCU GearBoxIn rotv_out"
  Demux/6 -> BusCreator/6  "TCU GearBoxIn Trq_in"
  Demux/7 -> BusCreator/7  "TCU GearBoxIn Trq_out"
  Demux/8 -> BusCreator/8  "TCU GearBoxIn Trq_out_trg"
  Demux/9 -> BusCreator/9  "TCU GearBoxIn Clutch rotv_in"
  Demux/10 -> BusCreator/10  "TCU GearBoxIn Clutch rotv_out"
  Demux/11 -> BusCreator/11  "TCU GearBoxIn Clutch rotv_out_trg"
  Demux/12 -> BusCreator/12  "TCU GearBoxIn Clutch Trq_in"
  Demux/13 -> BusCreator/13  "TCU GearBoxIn Clutch Trq_out"
  Demux/14 -> BusCreator/14  "TCU GearBoxIn Clutch Trq_out_trg"
  Demux/15 -> BusCreator/15  "TCU GearBoxIn Clutch i_TrqIn2Out"

== system PTTransmCU/CarMaker/IPG Vehicle/PowerTrain/TCU Example/PTTransmCU_In/CreateBus TCU GearBoxM_In0 ==
  In : Inport
  BusCreator : BusCreator  Inputs=15
  Demux : Demux  Outputs=15
  Out : Outport
  wires:
  In/1 -> Demux/1
  BusCreator/1 -> Out/1
  Demux/1 -> BusCreator/1  "TCU GearBoxM_In0 GearNo"
  Demux/2 -> BusCreator/2  "TCU GearBoxM_In0 i"
  Demux/3 -> BusCreator/3  "TCU GearBoxM_In0 rotv_in"
  Demux/4 -> BusCreator/4  "TCU GearBoxM_In0 rotv_in_trg"
  Demux/5 -> BusCreator/5  "TCU GearBoxM_In0 rotv_out"
  Demux/6 -> BusCreator/6  "TCU GearBoxM_In0 Trq_in"
  Demux/7 -> BusCreator/7  "TCU GearBoxM_In0 Trq_out"
  Demux/8 -> BusCreator/8  "TCU GearBoxM_In0 Trq_out_trg"
  Demux/9 -> BusCreator/9  "TCU GearBoxM_In0 Clutch rotv_in"
  Demux/10 -> BusCreator/10  "TCU GearBoxM_In0 Clutch rotv_out"
  Demux/11 -> BusCreator/11  "TCU GearBoxM_In0 Clutch rotv_out_trg"
  Demux/12 -> BusCreator/12  "TCU GearBoxM_In0 Clutch Trq_in"
  Demux/13 -> BusCreator/13  "TCU GearBoxM_In0 Clutch Trq_out"
  Demux/14 -> BusCreator/14  "TCU GearBoxM_In0 Clutch Trq_out_trg"
  Demux/15 -> BusCreator/15  "TCU GearBoxM_In0 Clutch i_TrqIn2Out"

== system PTTransmCU/CarMaker/IPG Vehicle/PowerTrain/TCU Example/PTTransmCU_In/CreateBus TCU GearBoxM_In1 ==
  In : Inport
  BusCreator : BusCreator  Inputs=15
  Demux : Demux  Outputs=15
  Out : Outport
  wires:
  In/1 -> Demux/1
  BusCreator/1 -> Out/1
  Demux/1 -> BusCreator/1  "TCU GearBoxM_In1 GearNo"
  Demux/2 -> BusCreator/2  "TCU GearBoxM_In1 i"
  Demux/3 -> BusCreator/3  "TCU GearBoxM_In1 rotv_in"
  Demux/4 -> BusCreator/4  "TCU GearBoxM_In1 rotv_in_trg"
  Demux/5 -> BusCreator/5  "TCU GearBoxM_In1 rotv_out"
  Demux/6 -> BusCreator/6  "TCU GearBoxM_In1 Trq_in"
  Demux/7 -> BusCreator/7  "TCU GearBoxM_In1 Trq_out"
  Demux/8 -> BusCreator/8  "TCU GearBoxM_In1 Trq_out_trg"
  Demux/9 -> BusCreator/9  "TCU GearBoxM_In1 Clutch rotv_in"
  Demux/10 -> BusCreator/10  "TCU GearBoxM_In1 Clutch rotv_out"
  Demux/11 -> BusCreator/11  "TCU GearBoxM_In1 Clutch rotv_out_trg"
  Demux/12 -> BusCreator/12  "TCU GearBoxM_In1 Clutch Trq_in"
  Demux/13 -> BusCreator/13  "TCU GearBoxM_In1 Clutch Trq_out"
  Demux/14 -> BusCreator/14  "TCU GearBoxM_In1 Clutch Trq_out_trg"
  Demux/15 -> BusCreator/15  "TCU GearBoxM_In1 Clutch i_TrqIn2Out"

== system PTTransmCU/CarMaker/IPG Vehicle/PowerTrain/TCU Example/PTTransmCU_In/CreateBus TCU GearBoxM_In2 ==
  In : Inport
  BusCreator : BusCreator  Inputs=15
  Demux : Demux  Outputs=15
  Out : Outport
  wires:
  In/1 -> Demux/1
  BusCreator/1 -> Out/1
  Demux/1 -> BusCreator/1  "TCU GearBoxM_In2 GearNo"
  Demux/2 -> BusCreator/2  "TCU GearBoxM_In2 i"
  Demux/3 -> BusCreator/3  "TCU GearBoxM_In2 rotv_in"
  Demux/4 -> BusCreator/4  "TCU GearBoxM_In2 rotv_in_trg"
  Demux/5 -> BusCreator/5  "TCU GearBoxM_In2 rotv_out"
  Demux/6 -> BusCreator/6  "TCU GearBoxM_In2 Trq_in"
  Demux/7 -> BusCreator/7  "TCU GearBoxM_In2 Trq_out"
  Demux/8 -> BusCreator/8  "TCU GearBoxM_In2 Trq_out_trg"
  Demux/9 -> BusCreator/9  "TCU GearBoxM_In2 Clutch rotv_in"
  Demux/10 -> BusCreator/10  "TCU GearBoxM_In2 Clutch rotv_out"
  Demux/11 -> BusCreator/11  "TCU GearBoxM_In2 Clutch rotv_out_trg"
  Demux/12 -> BusCreator/12  "TCU GearBoxM_In2 Clutch Trq_in"
  Demux/13 -> BusCreator/13  "TCU GearBoxM_In2 Clutch Trq_out"
  Demux/14 -> BusCreator/14  "TCU GearBoxM_In2 Clutch Trq_out_trg"
  Demux/15 -> BusCreator/15  "TCU GearBoxM_In2 Clutch i_TrqIn2Out"

== system PTTransmCU/CarMaker/IPG Vehicle/PowerTrain/TCU Example/PTTransmCU_In/CreateBus TCU GearBoxM_In3 ==
  In : Inport
  BusCreator : BusCreator  Inputs=15
  Demux : Demux  Outputs=15
  Out : Outport
  wires:
  In/1 -> Demux/1
  BusCreator/1 -> Out/1
  Demux/1 -> BusCreator/1  "TCU GearBoxM_In3 GearNo"
  Demux/2 -> BusCreator/2  "TCU GearBoxM_In3 i"
  Demux/3 -> BusCreator/3  "TCU GearBoxM_In3 rotv_in"
  Demux/4 -> BusCreator/4  "TCU GearBoxM_In3 rotv_in_trg"
  Demux/5 -> BusCreator/5  "TCU GearBoxM_In3 rotv_out"
  Demux/6 -> BusCreator/6  "TCU GearBoxM_In3 Trq_in"
  Demux/7 -> BusCreator/7  "TCU GearBoxM_In3 Trq_out"
  Demux/8 -> BusCreator/8  "TCU GearBoxM_In3 Trq_out_trg"
  Demux/9 -> BusCreator/9  "TCU GearBoxM_In3 Clutch rotv_in"
  Demux/10 -> BusCreator/10  "TCU GearBoxM_In3 Clutch rotv_out"
  Demux/11 -> BusCreator/11  "TCU GearBoxM_In3 Clutch rotv_out_trg"
  Demux/12 -> BusCreator/12  "TCU GearBoxM_In3 Clutch Trq_in"
  Demux/13 -> BusCreator/13  "TCU GearBoxM_In3 Clutch Trq_out"
  Demux/14 -> BusCreator/14  "TCU GearBoxM_In3 Clutch Trq_out_trg"
  Demux/15 -> BusCreator/15  "TCU GearBoxM_In3 Clutch i_TrqIn2Out"

== system PTTransmCU/CarMaker/IPG Vehicle/PowerTrain/TCU Example/PTTransmCU_In/CreateBus TCU GearBoxM_Out0 ==
  In : Inport
  BusCreator : BusCreator  Inputs=3
  Demux : Demux  Outputs=3
  Out : Outport
  wires:
  In/1 -> Demux/1
  BusCreator/1 -> Out/1
  Demux/1 -> BusCreator/1  "TCU GearBoxM_Out0 GearNoTrg"
  Demux/2 -> BusCreator/2  "TCU GearBoxM_Out0 set_ParkBrake"
  Demux/3 -> BusCreator/3  "TCU GearBoxM_Out0 Clutch Pos"

== system PTTransmCU/CarMaker/IPG Vehicle/PowerTrain/TCU Example/PTTransmCU_In/CreateBus TCU GearBoxM_Out1 ==
  In : Inport
  BusCreator : BusCreator  Inputs=3
  Demux : Demux  Outputs=3
  Out : Outport
  wires:
  In/1 -> Demux/1
  BusCreator/1 -> Out/1
  Demux/1 -> BusCreator/1  "TCU GearBoxM_Out1 GearNoTrg"
  Demux/2 -> BusCreator/2  "TCU GearBoxM_Out1 set_ParkBrake"
  Demux/3 -> BusCreator/3  "TCU GearBoxM_Out1 Clutch Pos"

== system PTTransmCU/CarMaker/IPG Vehicle/PowerTrain/TCU Example/PTTransmCU_In/CreateBus TCU GearBoxM_Out2 ==
  In : Inport
  BusCreator : BusCreator  Inputs=3
  Demux : Demux  Outputs=3
  Out : Outport
  wires:
  In/1 -> Demux/1
  BusCreator/1 -> Out/1
  Demux/1 -> BusCreator/1  "TCU GearBoxM_Out2 GearNoTrg"
  Demux/2 -> BusCreator/2  "TCU GearBoxM_Out2 set_ParkBrake"
  Demux/3 -> BusCreator/3  "TCU GearBoxM_Out2 Clutch Pos"

== system PTTransmCU/CarMaker/IPG Vehicle/PowerTrain/TCU Example/PTTransmCU_In/CreateBus TCU GearBoxM_Out3 ==
  In : Inport
  BusCreator : BusCreator  Inputs=3
  Demux : Demux  Outputs=3
  Out : Outport
  wires:
  In/1 -> Demux/1
  BusCreator/1 -> Out/1
  Demux/1 -> BusCreator/1  "TCU GearBoxM_Out3 GearNoTrg"
  Demux/2 -> BusCreator/2  "TCU GearBoxM_Out3 set_ParkBrake"
  Demux/3 -> BusCreator/3  "TCU GearBoxM_Out3 Clutch Pos"

== system PTTransmCU/CarMaker/IPG Vehicle/PowerTrain/TCU Example/PTTransmCU_In/CreateBus TCU GearBoxOut ==
  In : Inport
  BusCreator : BusCreator  Inputs=3
  Demux : Demux  Outputs=3
  Out : Outport
  wires:
  In/1 -> Demux/1
  BusCreator/1 -> Out/1
  Demux/1 -> BusCreator/1  "TCU GearBoxIn GearNoTrg"
  Demux/2 -> BusCreator/2  "TCU GearBoxIn set_ParkBrake"
  Demux/3 -> BusCreator/3  "TCU GearBoxIn Clutch Pos"

== system PTTransmCU/CarMaker/IPG Vehicle/PowerTrain/TCU Example/PTTransmCU_In/CreateBus TCU Input ==
  In : Inport
  BusCreator : BusCreator  Inputs=3
  Demux : Demux  Outputs=3
  Out : Outport
  wires:
  In/1 -> Demux/1
  BusCreator/1 -> Out/1
  Demux/1 -> BusCreator/1  "TCU Ignition"
  Demux/2 -> BusCreator/2  "TCU Load"
  Demux/3 -> BusCreator/3  "TCU SelectorCtrl"

== system PTTransmCU/CarMaker/IPG Vehicle/PowerTrain/TCU Example/PTTransmCU_In/CreateBus TCU_Cfg GearBox ==
  In : Inport
  BusCreator : BusCreator  Inputs=38
  Demux : Demux  Outputs=38
  Out : Outport
  wires:
  In/1 -> Demux/1
  BusCreator/1 -> Out/1
  Demux/1 -> BusCreator/1  "TCU_Cfg GearBox GBKind"
  Demux/2 -> BusCreator/2  "TCU_Cfg GearBox ClKind"
  Demux/3 -> BusCreator/3  "TCU_Cfg GearBox nFGears"
  Demux/4 -> BusCreator/4  "TCU_Cfg GearBox iFGear0"
  Demux/5 -> BusCreator/5  "TCU_Cfg GearBox iFGear1"
  Demux/6 -> BusCreator/6  "TCU_Cfg GearBox iFGear2"
  Demux/7 -> BusCreator/7  "TCU_Cfg GearBox iFGear3"
  Demux/8 -> BusCreator/8  "TCU_Cfg GearBox iFGear4"
  Demux/9 -> BusCreator/9  "TCU_Cfg GearBox iFGear5"
  Demux/10 -> BusCreator/10  "TCU_Cfg GearBox iFGear6"
  Demux/11 -> BusCreator/11  "TCU_Cfg GearBox iFGear7"
  Demux/12 -> BusCreator/12  "TCU_Cfg GearBox iFGear8"
  Demux/13 -> BusCreator/13  "TCU_Cfg GearBox iFGear9"
  Demux/14 -> BusCreator/14  "TCU_Cfg GearBox iFGear10"
  Demux/15 -> BusCreator/15  "TCU_Cfg GearBox iFGear11"
  Demux/16 -> BusCreator/16  "TCU_Cfg GearBox iFGear12"
  Demux/17 -> BusCreator/17  "TCU_Cfg GearBox iFGear13"
  Demux/18 -> BusCreator/18  "TCU_Cfg GearBox iFGear14"
  Demux/19 -> BusCreator/19  "TCU_Cfg GearBox iFGear15"
  Demux/20 -> BusCreator/20  "TCU_Cfg GearBox iFGear16"
  Demux/21 -> BusCreator/21  "TCU_Cfg GearBox nBGears"
  Demux/22 -> BusCreator/22  "TCU_Cfg GearBox iBGear0"
  Demux/23 -> BusCreator/23  "TCU_Cfg GearBox iBGear1"
  Demux/24 -> BusCreator/24  "TCU_Cfg GearBox iBGear2"
  Demux/25 -> BusCreator/25  "TCU_Cfg GearBox iBGear3"
  Demux/26 -> BusCreator/26  "TCU_Cfg GearBox iBGear4"
  Demux/27 -> BusCreator/27  "TCU_Cfg GearBox iBGear5"
  Demux/28 -> BusCreator/28  "TCU_Cfg GearBox iBGear6"
  Demux/29 -> BusCreator/29  "TCU_Cfg GearBox iBGear7"
  Demux/30 -> BusCreator/30  "TCU_Cfg GearBox iBGear8"
  Demux/31 -> BusCreator/31  "TCU_Cfg GearBox iBGear9"
  Demux/32 -> BusCreator/32  "TCU_Cfg GearBox iBGear10"
  Demux/33 -> BusCreator/33  "TCU_Cfg GearBox iBGear11"
  Demux/34 -> BusCreator/34  "TCU_Cfg GearBox iBGear12"
  Demux/35 -> BusCreator/35  "TCU_Cfg GearBox iBGear13"
  Demux/36 -> BusCreator/36  "TCU_Cfg GearBox iBGear14"
  Demux/37 -> BusCreator/37  "TCU_Cfg GearBox iBGear15"
  Demux/38 -> BusCreator/38  "TCU_Cfg GearBox iBGear16"

== system PTTransmCU/CarMaker/IPG Vehicle/PowerTrain/TCU Example/PTTransmCU_In/CreateBus TCU_Cfg GearBoxM0 ==
  In : Inport
  BusCreator : BusCreator  Inputs=38
  Demux : Demux  Outputs=38
  Out : Outport
  wires:
  In/1 -> Demux/1
  BusCreator/1 -> Out/1
  Demux/1 -> BusCreator/1  "TCU_Cfg GearBoxM0 GBKind"
  Demux/2 -> BusCreator/2  "TCU_Cfg GearBoxM0 ClKind"
  Demux/3 -> BusCreator/3  "TCU_Cfg GearBoxM0 nFGears"
  Demux/4 -> BusCreator/4  "TCU_Cfg GearBoxM0 iFGear0"
  Demux/5 -> BusCreator/5  "TCU_Cfg GearBoxM0 iFGear1"
  Demux/6 -> BusCreator/6  "TCU_Cfg GearBoxM0 iFGear2"
  Demux/7 -> BusCreator/7  "TCU_Cfg GearBoxM0 iFGear3"
  Demux/8 -> BusCreator/8  "TCU_Cfg GearBoxM0 iFGear4"
  Demux/9 -> BusCreator/9  "TCU_Cfg GearBoxM0 iFGear5"
  Demux/10 -> BusCreator/10  "TCU_Cfg GearBoxM0 iFGear6"
  Demux/11 -> BusCreator/11  "TCU_Cfg GearBoxM0 iFGear7"
  Demux/12 -> BusCreator/12  "TCU_Cfg GearBoxM0 iFGear8"
  Demux/13 -> BusCreator/13  "TCU_Cfg GearBoxM0 iFGear9"
  Demux/14 -> BusCreator/14  "TCU_Cfg GearBoxM0 iFGear10"
  Demux/15 -> BusCreator/15  "TCU_Cfg GearBoxM0 iFGear11"
  Demux/16 -> BusCreator/16  "TCU_Cfg GearBoxM0 iFGear12"
  Demux/17 -> BusCreator/17  "TCU_Cfg GearBoxM0 iFGear13"
  Demux/18 -> BusCreator/18  "TCU_Cfg GearBoxM0 iFGear14"
  Demux/19 -> BusCreator/19  "TCU_Cfg GearBoxM0 iFGear15"
  Demux/20 -> BusCreator/20  "TCU_Cfg GearBoxM0 iFGear16"
  Demux/21 -> BusCreator/21  "TCU_Cfg GearBoxM0 nBGears"
  Demux/22 -> BusCreator/22  "TCU_Cfg GearBoxM0 iBGear0"
  Demux/23 -> BusCreator/23  "TCU_Cfg GearBoxM0 iBGear1"
  Demux/24 -> BusCreator/24  "TCU_Cfg GearBoxM0 iBGear2"
  Demux/25 -> BusCreator/25  "TCU_Cfg GearBoxM0 iBGear3"
  Demux/26 -> BusCreator/26  "TCU_Cfg GearBoxM0 iBGear4"
  Demux/27 -> BusCreator/27  "TCU_Cfg GearBoxM0 iBGear5"
  Demux/28 -> BusCreator/28  "TCU_Cfg GearBoxM0 iBGear6"
  Demux/29 -> BusCreator/29  "TCU_Cfg GearBoxM0 iBGear7"
  Demux/30 -> BusCreator/30  "TCU_Cfg GearBoxM0 iBGear8"
  Demux/31 -> BusCreator/31  "TCU_Cfg GearBoxM0 iBGear9"
  Demux/32 -> BusCreator/32  "TCU_Cfg GearBoxM0 iBGear10"
  Demux/33 -> BusCreator/33  "TCU_Cfg GearBoxM0 iBGear11"
  Demux/34 -> BusCreator/34  "TCU_Cfg GearBoxM0 iBGear12"
  Demux/35 -> BusCreator/35  "TCU_Cfg GearBoxM0 iBGear13"
  Demux/36 -> BusCreator/36  "TCU_Cfg GearBoxM0 iBGear14"
  Demux/37 -> BusCreator/37  "TCU_Cfg GearBoxM0 iBGear15"
  Demux/38 -> BusCreator/38  "TCU_Cfg GearBoxM0 iBGear16"

== system PTTransmCU/CarMaker/IPG Vehicle/PowerTrain/TCU Example/PTTransmCU_In/CreateBus TCU_Cfg GearBoxM1 ==
  In : Inport
  BusCreator : BusCreator  Inputs=38
  Demux : Demux  Outputs=38
  Out : Outport
  wires:
  In/1 -> Demux/1
  BusCreator/1 -> Out/1
  Demux/1 -> BusCreator/1  "TCU_Cfg GearBoxM1 GBKind"
  Demux/2 -> BusCreator/2  "TCU_Cfg GearBoxM1 ClKind"
  Demux/3 -> BusCreator/3  "TCU_Cfg GearBoxM1 nFGears"
  Demux/4 -> BusCreator/4  "TCU_Cfg GearBoxM1 iFGear0"
  Demux/5 -> BusCreator/5  "TCU_Cfg GearBoxM1 iFGear1"
  Demux/6 -> BusCreator/6  "TCU_Cfg GearBoxM1 iFGear2"
  Demux/7 -> BusCreator/7  "TCU_Cfg GearBoxM1 iFGear3"
  Demux/8 -> BusCreator/8  "TCU_Cfg GearBoxM1 iFGear4"
  Demux/9 -> BusCreator/9  "TCU_Cfg GearBoxM1 iFGear5"
  Demux/10 -> BusCreator/10  "TCU_Cfg GearBoxM1 iFGear6"
  Demux/11 -> BusCreator/11  "TCU_Cfg GearBoxM1 iFGear7"
  Demux/12 -> BusCreator/12  "TCU_Cfg GearBoxM1 iFGear8"
  Demux/13 -> BusCreator/13  "TCU_Cfg GearBoxM1 iFGear9"
  Demux/14 -> BusCreator/14  "TCU_Cfg GearBoxM1 iFGear10"
  Demux/15 -> BusCreator/15  "TCU_Cfg GearBoxM1 iFGear11"
  Demux/16 -> BusCreator/16  "TCU_Cfg GearBoxM1 iFGear12"
  Demux/17 -> BusCreator/17  "TCU_Cfg GearBoxM1 iFGear13"
  Demux/18 -> BusCreator/18  "TCU_Cfg GearBoxM1 iFGear14"
  Demux/19 -> BusCreator/19  "TCU_Cfg GearBoxM1 iFGear15"
  Demux/20 -> BusCreator/20  "TCU_Cfg GearBoxM1 iFGear16"
  Demux/21 -> BusCreator/21  "TCU_Cfg GearBoxM1 nBGears"
  Demux/22 -> BusCreator/22  "TCU_Cfg GearBoxM1 iBGear0"
  Demux/23 -> BusCreator/23  "TCU_Cfg GearBoxM1 iBGear1"
  Demux/24 -> BusCreator/24  "TCU_Cfg GearBoxM1 iBGear2"
  Demux/25 -> BusCreator/25  "TCU_Cfg GearBoxM1 iBGear3"
  Demux/26 -> BusCreator/26  "TCU_Cfg GearBoxM1 iBGear4"
  Demux/27 -> BusCreator/27  "TCU_Cfg GearBoxM1 iBGear5"
  Demux/28 -> BusCreator/28  "TCU_Cfg GearBoxM1 iBGear6"
  Demux/29 -> BusCreator/29  "TCU_Cfg GearBoxM1 iBGear7"
  Demux/30 -> BusCreator/30  "TCU_Cfg GearBoxM1 iBGear8"
  Demux/31 -> BusCreator/31  "TCU_Cfg GearBoxM1 iBGear9"
  Demux/32 -> BusCreator/32  "TCU_Cfg GearBoxM1 iBGear10"
  Demux/33 -> BusCreator/33  "TCU_Cfg GearBoxM1 iBGear11"
  Demux/34 -> BusCreator/34  "TCU_Cfg GearBoxM1 iBGear12"
  Demux/35 -> BusCreator/35  "TCU_Cfg GearBoxM1 iBGear13"
  Demux/36 -> BusCreator/36  "TCU_Cfg GearBoxM1 iBGear14"
  Demux/37 -> BusCreator/37  "TCU_Cfg GearBoxM1 iBGear15"
  Demux/38 -> BusCreator/38  "TCU_Cfg GearBoxM1 iBGear16"

== system PTTransmCU/CarMaker/IPG Vehicle/PowerTrain/TCU Example/PTTransmCU_In/CreateBus TCU_Cfg GearBoxM2 ==
  In : Inport
  BusCreator : BusCreator  Inputs=38
  Demux : Demux  Outputs=38
  Out : Outport
  wires:
  In/1 -> Demux/1
  BusCreator/1 -> Out/1
  Demux/1 -> BusCreator/1  "TCU_Cfg GearBoxM2 GBKind"
  Demux/2 -> BusCreator/2  "TCU_Cfg GearBoxM2 ClKind"
  Demux/3 -> BusCreator/3  "TCU_Cfg GearBoxM2 nFGears"
  Demux/4 -> BusCreator/4  "TCU_Cfg GearBoxM2 iFGear0"
  Demux/5 -> BusCreator/5  "TCU_Cfg GearBoxM2 iFGear1"
  Demux/6 -> BusCreator/6  "TCU_Cfg GearBoxM2 iFGear2"
  Demux/7 -> BusCreator/7  "TCU_Cfg GearBoxM2 iFGear3"
  Demux/8 -> BusCreator/8  "TCU_Cfg GearBoxM2 iFGear4"
  Demux/9 -> BusCreator/9  "TCU_Cfg GearBoxM2 iFGear5"
  Demux/10 -> BusCreator/10  "TCU_Cfg GearBoxM2 iFGear6"
  Demux/11 -> BusCreator/11  "TCU_Cfg GearBoxM2 iFGear7"
  Demux/12 -> BusCreator/12  "TCU_Cfg GearBoxM2 iFGear8"
  Demux/13 -> BusCreator/13  "TCU_Cfg GearBoxM2 iFGear9"
  Demux/14 -> BusCreator/14  "TCU_Cfg GearBoxM2 iFGear10"
  Demux/15 -> BusCreator/15  "TCU_Cfg GearBoxM2 iFGear11"
  Demux/16 -> BusCreator/16  "TCU_Cfg GearBoxM2 iFGear12"
  Demux/17 -> BusCreator/17  "TCU_Cfg GearBoxM2 iFGear13"
  Demux/18 -> BusCreator/18  "TCU_Cfg GearBoxM2 iFGear14"
  Demux/19 -> BusCreator/19  "TCU_Cfg GearBoxM2 iFGear15"
  Demux/20 -> BusCreator/20  "TCU_Cfg GearBoxM2 iFGear16"
  Demux/21 -> BusCreator/21  "TCU_Cfg GearBoxM2 nBGears"
  Demux/22 -> BusCreator/22  "TCU_Cfg GearBoxM2 iBGear0"
  Demux/23 -> BusCreator/23  "TCU_Cfg GearBoxM2 iBGear1"
  Demux/24 -> BusCreator/24  "TCU_Cfg GearBoxM2 iBGear2"
  Demux/25 -> BusCreator/25  "TCU_Cfg GearBoxM2 iBGear3"
  Demux/26 -> BusCreator/26  "TCU_Cfg GearBoxM2 iBGear4"
  Demux/27 -> BusCreator/27  "TCU_Cfg GearBoxM2 iBGear5"
  Demux/28 -> BusCreator/28  "TCU_Cfg GearBoxM2 iBGear6"
  Demux/29 -> BusCreator/29  "TCU_Cfg GearBoxM2 iBGear7"
  Demux/30 -> BusCreator/30  "TCU_Cfg GearBoxM2 iBGear8"
  Demux/31 -> BusCreator/31  "TCU_Cfg GearBoxM2 iBGear9"
  Demux/32 -> BusCreator/32  "TCU_Cfg GearBoxM2 iBGear10"
  Demux/33 -> BusCreator/33  "TCU_Cfg GearBoxM2 iBGear11"
  Demux/34 -> BusCreator/34  "TCU_Cfg GearBoxM2 iBGear12"
  Demux/35 -> BusCreator/35  "TCU_Cfg GearBoxM2 iBGear13"
  Demux/36 -> BusCreator/36  "TCU_Cfg GearBoxM2 iBGear14"
  Demux/37 -> BusCreator/37  "TCU_Cfg GearBoxM2 iBGear15"
  Demux/38 -> BusCreator/38  "TCU_Cfg GearBoxM2 iBGear16"

== system PTTransmCU/CarMaker/IPG Vehicle/PowerTrain/TCU Example/PTTransmCU_In/CreateBus TCU_Cfg GearBoxM3 ==
  In : Inport
  BusCreator : BusCreator  Inputs=38
  Demux : Demux  Outputs=38
  Out : Outport
  wires:
  In/1 -> Demux/1
  BusCreator/1 -> Out/1
  Demux/1 -> BusCreator/1  "TCU_Cfg GearBoxM3 GBKind"
  Demux/2 -> BusCreator/2  "TCU_Cfg GearBoxM3 ClKind"
  Demux/3 -> BusCreator/3  "TCU_Cfg GearBoxM3 nFGears"
  Demux/4 -> BusCreator/4  "TCU_Cfg GearBoxM3 iFGear0"
  Demux/5 -> BusCreator/5  "TCU_Cfg GearBoxM3 iFGear1"
  Demux/6 -> BusCreator/6  "TCU_Cfg GearBoxM3 iFGear2"
  Demux/7 -> BusCreator/7  "TCU_Cfg GearBoxM3 iFGear3"
  Demux/8 -> BusCreator/8  "TCU_Cfg GearBoxM3 iFGear4"
  Demux/9 -> BusCreator/9  "TCU_Cfg GearBoxM3 iFGear5"
  Demux/10 -> BusCreator/10  "TCU_Cfg GearBoxM3 iFGear6"
  Demux/11 -> BusCreator/11  "TCU_Cfg GearBoxM3 iFGear7"
  Demux/12 -> BusCreator/12  "TCU_Cfg GearBoxM3 iFGear8"
  Demux/13 -> BusCreator/13  "TCU_Cfg GearBoxM3 iFGear9"
  Demux/14 -> BusCreator/14  "TCU_Cfg GearBoxM3 iFGear10"
  Demux/15 -> BusCreator/15  "TCU_Cfg GearBoxM3 iFGear11"
  Demux/16 -> BusCreator/16  "TCU_Cfg GearBoxM3 iFGear12"
  Demux/17 -> BusCreator/17  "TCU_Cfg GearBoxM3 iFGear13"
  Demux/18 -> BusCreator/18  "TCU_Cfg GearBoxM3 iFGear14"
  Demux/19 -> BusCreator/19  "TCU_Cfg GearBoxM3 iFGear15"
  Demux/20 -> BusCreator/20  "TCU_Cfg GearBoxM3 iFGear16"
  Demux/21 -> BusCreator/21  "TCU_Cfg GearBoxM3 nBGears"
  Demux/22 -> BusCreator/22  "TCU_Cfg GearBoxM3 iBGear0"
  Demux/23 -> BusCreator/23  "TCU_Cfg GearBoxM3 iBGear1"
  Demux/24 -> BusCreator/24  "TCU_Cfg GearBoxM3 iBGear2"
  Demux/25 -> BusCreator/25  "TCU_Cfg GearBoxM3 iBGear3"
  Demux/26 -> BusCreator/26  "TCU_Cfg GearBoxM3 iBGear4"
  Demux/27 -> BusCreator/27  "TCU_Cfg GearBoxM3 iBGear5"
  Demux/28 -> BusCreator/28  "TCU_Cfg GearBoxM3 iBGear6"
  Demux/29 -> BusCreator/29  "TCU_Cfg GearBoxM3 iBGear7"
  Demux/30 -> BusCreator/30  "TCU_Cfg GearBoxM3 iBGear8"
  Demux/31 -> BusCreator/31  "TCU_Cfg GearBoxM3 iBGear9"
  Demux/32 -> BusCreator/32  "TCU_Cfg GearBoxM3 iBGear10"
  Demux/33 -> BusCreator/33  "TCU_Cfg GearBoxM3 iBGear11"
  Demux/34 -> BusCreator/34  "TCU_Cfg GearBoxM3 iBGear12"
  Demux/35 -> BusCreator/35  "TCU_Cfg GearBoxM3 iBGear13"
  Demux/36 -> BusCreator/36  "TCU_Cfg GearBoxM3 iBGear14"
  Demux/37 -> BusCreator/37  "TCU_Cfg GearBoxM3 iBGear15"
  Demux/38 -> BusCreator/38  "TCU_Cfg GearBoxM3 iBGear16"
